simulink model "latest_coil"  (R2021b)
settings: Solver=FixedStepAuto  StartTime=-18e-3  StopTime=50e-3  FixedStep=1e-4  RelTol=1e-3
undefined symbols (not defined in the file): X, Y, Z
libraries: sm_lib x28, nesl_utility x9
(part 2 of 5)

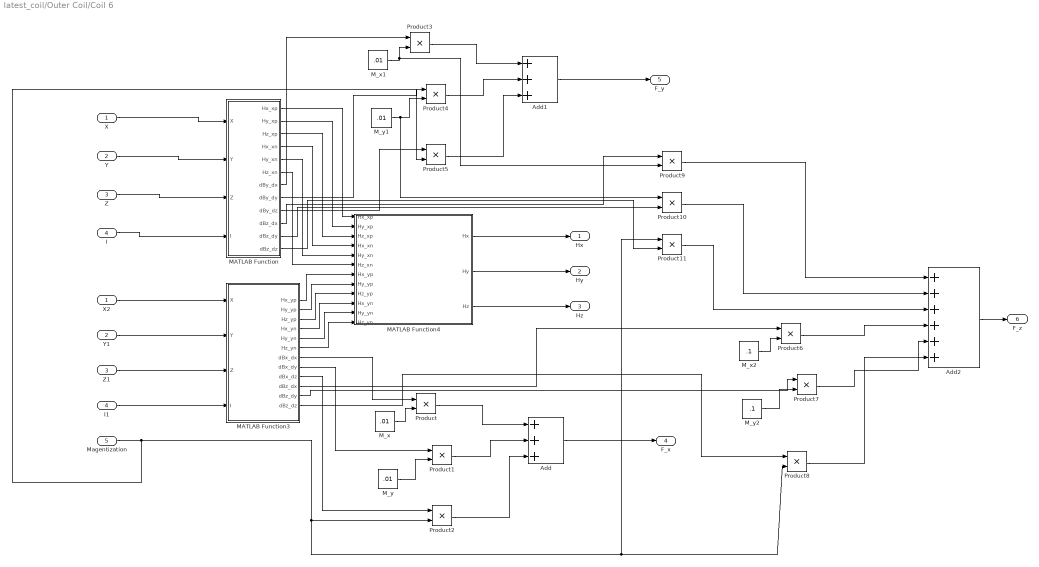
== system latest_coil/Outer Coil/Coil 6 ==
  X : Inport
  Y : Inport  Port=2
  Z : Inport  Port=3
  I : Inport  Port=4
  Magentization : Inport  Port=5
  Add : Sum  Inputs=+++
  Add1 : Sum  Inputs=+++
  Add2 : Sum  Inputs=++++++
  I1 : InportShadow  Port=4
  MATLAB Function : MATLAB Function  TreatAsAtomicUnit=on
  MATLAB Function3 : MATLAB Function  TreatAsAtomicUnit=on
  MATLAB Function4 : MATLAB Function  TreatAsAtomicUnit=on
  M_x : Constant  Value=.01
  M_x1 : Constant  Value=.01
  M_x2 : Constant  Value=.1
  M_y : Constant  Value=.01
  M_y1 : Constant  Value=.01
  M_y2 : Constant  Value=.1
  Product{,1..11} (12 alike) : Product
  X2 : InportShadow
  Y1 : InportShadow  Port=2
  Z1 : InportShadow  Port=3
  Hx : Outport
  Hy : Outport  Port=2
  Hz : Outport  Port=3
  F_x : Outport  Port=4
  F_y : Outport  Port=5
  F_z : Outport  Port=6
  wires:
  Add2/1 -> F_z/1
  Product11/1 -> Add2/3
  Product10/1 -> Add2/2
  Product9/1 -> Add2/1
  MATLAB Function/12(dBz_dz) -> Product11/2
  MATLAB Function/11(dBz_dy) -> Product10/2
  MATLAB Function/10(dBz_dx) -> Product9/1
  MATLAB Function/8(dBy_dy) -> Product4/1
  M_x1/1 -> Product3/2, Product9/2
  MATLAB Function3/12(dBz_dz) -> Product8/1
  Product8/1 -> Add2/6
  M_x2/1 -> Product6/2
  MATLAB Function3/10(dBz_dx) -> Product6/1
  MATLAB Function3/11(dBz_dy) -> Product7/1
  M_y2/1 -> Product7/2
  Product6/1 -> Add2/4
  Product7/1 -> Add2/5
  MATLAB Function/7(dBy_dx) -> Product3/1
  M_y1/1 -> Product4/2, Product10/1
  MATLAB Function/9(dBy_dz) -> Product5/1
  Magentization/1 -> Product5/2, Product8/2, Product11/1, Product2/2
  Product3/1 -> Add1/1
  Product4/1 -> Add1/2
  Product5/1 -> Add1/3
  Add1/1 -> F_y/1
  Add/1 -> F_x/1
  Product2/1 -> Add/3
  Product1/1 -> Add/2
  Product/1 -> Add/1
  MATLAB Function3/9(dBx_dz) -> Product2/1
  M_y/1 -> Product1/2
  MATLAB Function3/8(dBx_dy) -> Product1/1
  MATLAB Function3/7(dBx_dx) -> Product/1
  M_x/1 -> Product/2
  Z1/1 -> MATLAB Function3/3(Z)
  Y1/1 -> MATLAB Function3/2(Y)
  X2/1 -> MATLAB Function3/1(X)
  I/1 -> MATLAB Function/4(I)
  MATLAB Function/2(Hy_xp) -> MATLAB Function4/2(Hy_xp)
  MATLAB Function3/6(Hz_yn) -> MATLAB Function4/12(Hz_yn)
  MATLAB Function3/5(Hy_yn) -> MATLAB Function4/11(Hy_yn)
  MATLAB Function/5(Hy_xn) -> MATLAB Function4/5(Hy_xn)
  Y/1 -> MATLAB Function/2(Y)
  MATLAB Function3/2(Hy_yp) -> MATLAB Function4/8(Hy_yp)
  MATLAB Function/1(Hx_xp) -> MATLAB Function4/1(Hx_xp)
  MATLAB Function/4(Hx_xn) -> MATLAB Function4/4(Hx_xn)
  MATLAB Function3/3(Hz_yp) -> MATLAB Function4/9(Hz_yp)
  MATLAB Function3/4(Hx_yn) -> MATLAB Function4/10(Hx_yn)
  MATLAB Function3/1(Hx_yp) -> MATLAB Function4/7(Hx_yp)
  MATLAB Function4/2(Hy) -> Hy/1
  MATLAB Function/3(Hz_xp) -> MATLAB Function4/3(Hz_xp)
  Z/1 -> MATLAB Function/3(Z)
  MATLAB Function/6(Hz_xn) -> MATLAB Function4/6(Hz_xn)
  I1/1 -> MATLAB Function3/4(I)
  MATLAB Function4/1(Hx) -> Hx/1
  X/1 -> MATLAB Function/1(X)
  MATLAB Function4/3(Hz) -> Hz/1

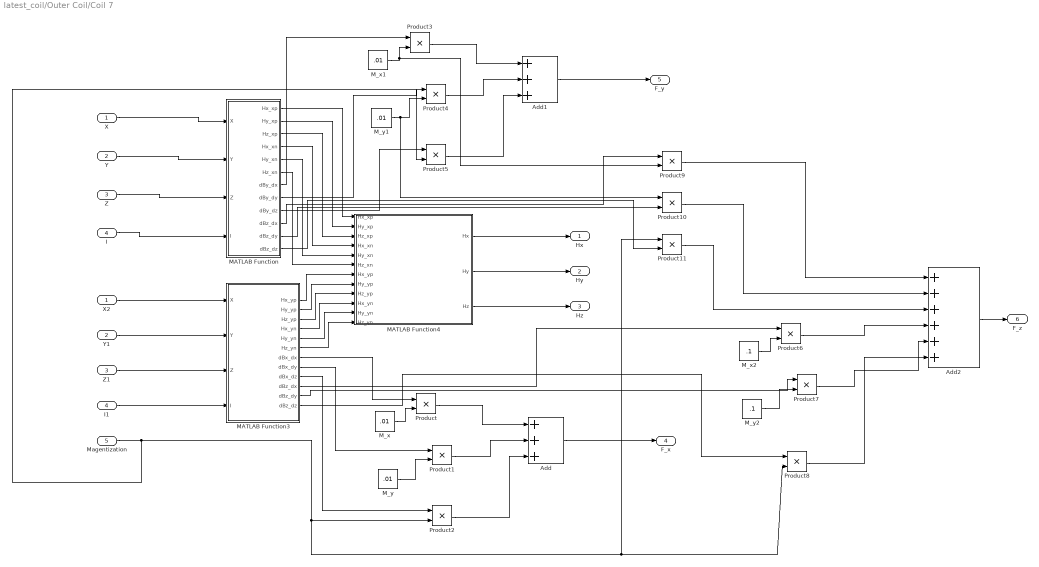
== system latest_coil/Outer Coil/Coil 7 ==
  X : Inport
  Y : Inport  Port=2
  Z : Inport  Port=3
  I : Inport  Port=4
  Magentization : Inport  Port=5
  Add : Sum  Inputs=+++
  Add1 : Sum  Inputs=+++
  Add2 : Sum  Inputs=++++++
  I1 : InportShadow  Port=4
  MATLAB Function : MATLAB Function  TreatAsAtomicUnit=on
  MATLAB Function3 : MATLAB Function  TreatAsAtomicUnit=on
  MATLAB Function4 : MATLAB Function  TreatAsAtomicUnit=on
  M_x : Constant  Value=.01
  M_x1 : Constant  Value=.01
  M_x2 : Constant  Value=.1
  M_y : Constant  Value=.01
  M_y1 : Constant  Value=.01
  M_y2 : Constant  Value=.1
  Product{,1..11} (12 alike) : Product
  X2 : InportShadow
  Y1 : InportShadow  Port=2
  Z1 : InportShadow  Port=3
  Hx : Outport
  Hy : Outport  Port=2
  Hz : Outport  Port=3
  F_x : Outport  Port=4
  F_y : Outport  Port=5
  F_z : Outport  Port=6
  wires:
  MATLAB Function4/3(Hz) -> Hz/1
  X/1 -> MATLAB Function/1(X)
  MATLAB Function4/1(Hx) -> Hx/1
  I1/1 -> MATLAB Function3/4(I)
  MATLAB Function/6(Hz_xn) -> MATLAB Function4/6(Hz_xn)
  Z/1 -> MATLAB Function/3(Z)
  MATLAB Function/3(Hz_xp) -> MATLAB Function4/3(Hz_xp)
  MATLAB Function4/2(Hy) -> Hy/1
  MATLAB Function3/1(Hx_yp) -> MATLAB Function4/7(Hx_yp)
  MATLAB Function3/4(Hx_yn) -> MATLAB Function4/10(Hx_yn)
  MATLAB Function3/3(Hz_yp) -> MATLAB Function4/9(Hz_yp)
  MATLAB Function/4(Hx_xn) -> MATLAB Function4/4(Hx_xn)
  MATLAB Function/1(Hx_xp) -> MATLAB Function4/1(Hx_xp)
  MATLAB Function3/2(Hy_yp) -> MATLAB Function4/8(Hy_yp)
  Y/1 -> MATLAB Function/2(Y)
  MATLAB Function/5(Hy_xn) -> MATLAB Function4/5(Hy_xn)
  MATLAB Function3/5(Hy_yn) -> MATLAB Function4/11(Hy_yn)
  MATLAB Function3/6(Hz_yn) -> MATLAB Function4/12(Hz_yn)
  MATLAB Function/2(Hy_xp) -> MATLAB Function4/2(Hy_xp)
  I/1 -> MATLAB Function/4(I)
  X2/1 -> MATLAB Function3/1(X)
  Y1/1 -> MATLAB Function3/2(Y)
  Z1/1 -> MATLAB Function3/3(Z)
  M_x/1 -> Product/2
  MATLAB Function3/7(dBx_dx) -> Product/1
  MATLAB Function3/8(dBx_dy) -> Product1/1
  M_y/1 -> Product1/2
  MATLAB Function3/9(dBx_dz) -> Product2/1
  Product/1 -> Add/1
  Product1/1 -> Add/2
  Product2/1 -> Add/3
  Add/1 -> F_x/1
  Add1/1 -> F_y/1
  Product5/1 -> Add1/3
  Product4/1 -> Add1/2
  Product3/1 -> Add1/1
  Magentization/1 -> Product2/2, Product11/1, Product8/2, Product5/2
  MATLAB Function/9(dBy_dz) -> Product5/1
  M_y1/1 -> Product10/1, Product4/2
  MATLAB Function/7(dBy_dx) -> Product3/1
  Product7/1 -> Add2/5
  Product6/1 -> Add2/4
  M_y2/1 -> Product7/2
  MATLAB Function3/11(dBz_dy) -> Product7/1
  MATLAB Function3/10(dBz_dx) -> Product6/1
  M_x2/1 -> Product6/2
  Product8/1 -> Add2/6
  MATLAB Function3/12(dBz_dz) -> Product8/1
  M_x1/1 -> Product9/2, Product3/2
  MATLAB Function/8(dBy_dy) -> Product4/1
  MATLAB Function/10(dBz_dx) -> Product9/1
  MATLAB Function/11(dBz_dy) -> Product10/2
  MATLAB Function/12(dBz_dz) -> Product11/2
  Product9/1 -> Add2/1
  Product10/1 -> Add2/2
  Product11/1 -> Add2/3
  Add2/1 -> F_z/1

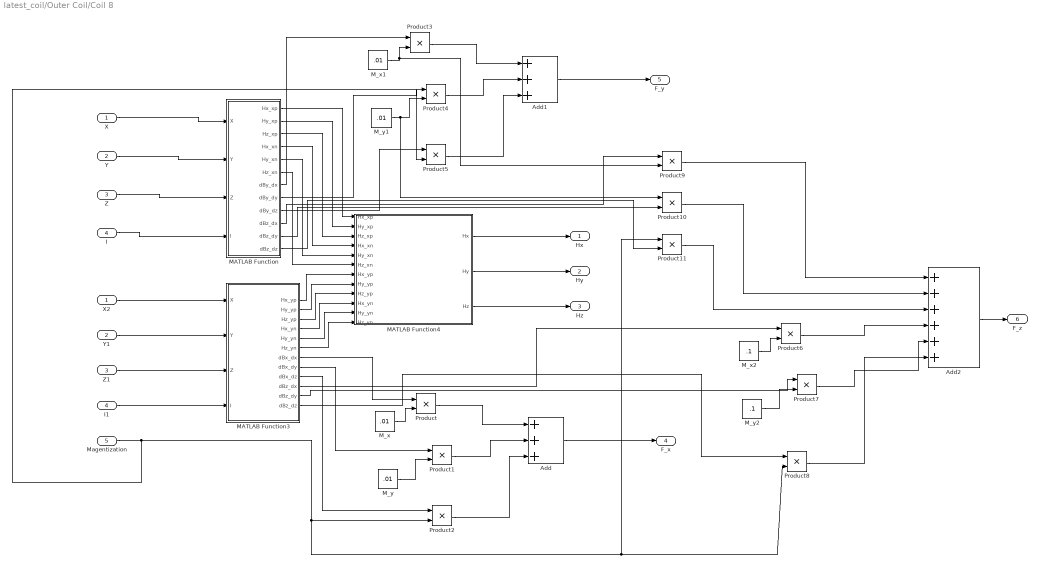
== system latest_coil/Outer Coil/Coil 8 ==
  X : Inport
  Y : Inport  Port=2
  Z : Inport  Port=3
  I : Inport  Port=4
  Magentization : Inport  Port=5
  Add : Sum  Inputs=+++
  Add1 : Sum  Inputs=+++
  Add2 : Sum  Inputs=++++++
  I1 : InportShadow  Port=4
  MATLAB Function : MATLAB Function  TreatAsAtomicUnit=on
  MATLAB Function3 : MATLAB Function  TreatAsAtomicUnit=on
  MATLAB Function4 : MATLAB Function  TreatAsAtomicUnit=on
  M_x : Constant  Value=.01
  M_x1 : Constant  Value=.01
  M_x2 : Constant  Value=.1
  M_y : Constant  Value=.01
  M_y1 : Constant  Value=.01
  M_y2 : Constant  Value=.1
  Product{,1..11} (12 alike) : Product
  X2 : InportShadow
  Y1 : InportShadow  Port=2
  Z1 : InportShadow  Port=3
  Hx : Outport
  Hy : Outport  Port=2
  Hz : Outport  Port=3
  F_x : Outport  Port=4
  F_y : Outport  Port=5
  F_z : Outport  Port=6
  wires:
  MATLAB Function4/3(Hz) -> Hz/1
  X/1 -> MATLAB Function/1(X)
  MATLAB Function4/1(Hx) -> Hx/1
  I1/1 -> MATLAB Function3/4(I)
  MATLAB Function/6(Hz_xn) -> MATLAB Function4/6(Hz_xn)
  Z/1 -> MATLAB Function/3(Z)
  MATLAB Function/3(Hz_xp) -> MATLAB Function4/3(Hz_xp)
  MATLAB Function4/2(Hy) -> Hy/1
  MATLAB Function3/1(Hx_yp) -> MATLAB Function4/7(Hx_yp)
  MATLAB Function3/4(Hx_yn) -> MATLAB Function4/10(Hx_yn)
  MATLAB Function3/3(Hz_yp) -> MATLAB Function4/9(Hz_yp)
  MATLAB Function/4(Hx_xn) -> MATLAB Function4/4(Hx_xn)
  MATLAB Function/1(Hx_xp) -> MATLAB Function4/1(Hx_xp)
  MATLAB Function3/2(Hy_yp) -> MATLAB Function4/8(Hy_yp)
  Y/1 -> MATLAB Function/2(Y)
  MATLAB Function/5(Hy_xn) -> MATLAB Function4/5(Hy_xn)
  MATLAB Function3/5(Hy_yn) -> MATLAB Function4/11(Hy_yn)
  MATLAB Function3/6(Hz_yn) -> MATLAB Function4/12(Hz_yn)
  MATLAB Function/2(Hy_xp) -> MATLAB Function4/2(Hy_xp)
  I/1 -> MATLAB Function/4(I)
  X2/1 -> MATLAB Function3/1(X)
  Y1/1 -> MATLAB Function3/2(Y)
  Z1/1 -> MATLAB Function3/3(Z)
  M_x/1 -> Product/2
  MATLAB Function3/7(dBx_dx) -> Product/1
  MATLAB Function3/8(dBx_dy) -> Product1/1
  M_y/1 -> Product1/2
  MATLAB Function3/9(dBx_dz) -> Product2/1
  Product/1 -> Add/1
  Product1/1 -> Add/2
  Product2/1 -> Add/3
  Add/1 -> F_x/1
  Add1/1 -> F_y/1
  Product5/1 -> Add1/3
  Product4/1 -> Add1/2
  Product3/1 -> Add1/1
  Magentization/1 -> Product2/2, Product11/1, Product8/2, Product5/2
  MATLAB Function/9(dBy_dz) -> Product5/1
  M_y1/1 -> Product10/1, Product4/2
  MATLAB Function/7(dBy_dx) -> Product3/1
  Product7/1 -> Add2/5
  Product6/1 -> Add2/4
  M_y2/1 -> Product7/2
  MATLAB Function3/11(dBz_dy) -> Product7/1
  MATLAB Function3/10(dBz_dx) -> Product6/1
  M_x2/1 -> Product6/2
  Product8/1 -> Add2/6
  MATLAB Function3/12(dBz_dz) -> Product8/1
  M_x1/1 -> Product9/2, Product3/2
  MATLAB Function/8(dBy_dy) -> Product4/1
  MATLAB Function/10(dBz_dx) -> Product9/1
  MATLAB Function/11(dBz_dy) -> Product10/2
  MATLAB Function/12(dBz_dz) -> Product11/2
  Product9/1 -> Add2/1
  Product10/1 -> Add2/2
  Product11/1 -> Add2/3
  Add2/1 -> F_z/1

== system latest_coil/Outer Coil/Coil 9 ==
  X : Inport
  Y : Inport  Port=2
  Z : Inport  Port=3
  I : Inport  Port=4
  Magentization : Inport  Port=5
  Add : Sum  Inputs=+++
  Add1 : Sum  Inputs=+++
  Add2 : Sum  Inputs=++++++
  I1 : InportShadow  Port=4
  MATLAB Function : MATLAB Function  TreatAsAtomicUnit=on
  MATLAB Function3 : MATLAB Function  TreatAsAtomicUnit=on
  MATLAB Function4 : MATLAB Function  TreatAsAtomicUnit=on
  M_x : Constant  Value=.01
  M_x1 : Constant  Value=.01
  M_x2 : Constant  Value=.1
  M_y : Constant  Value=.01
  M_y1 : Constant  Value=.01
  M_y2 : Constant  Value=.1
  Product{,1..11} (12 alike) : Product
  X2 : InportShadow
  Y1 : InportShadow  Port=2
  Z1 : InportShadow  Port=3
  Hx : Outport
  Hy : Outport  Port=2
  Hz : Outport  Port=3
  F_x : Outport  Port=4
  F_y : Outport  Port=5
  F_z : Outport  Port=6
  wires:
  Add2/1 -> F_z/1
  Product11/1 -> Add2/3
  Product10/1 -> Add2/2
  Product9/1 -> Add2/1
  MATLAB Function/12(dBz_dz) -> Product11/2
  MATLAB Function/11(dBz_dy) -> Product10/2
  MATLAB Function/10(dBz_dx) -> Product9/1
  MATLAB Function/8(dBy_dy) -> Product4/1
  M_x1/1 -> Product3/2, Product9/2
  MATLAB Function3/12(dBz_dz) -> Product8/1
  Product8/1 -> Add2/6
  M_x2/1 -> Product6/2
  MATLAB Function3/10(dBz_dx) -> Product6/1
  MATLAB Function3/11(dBz_dy) -> Product7/1
  M_y2/1 -> Product7/2
  Product6/1 -> Add2/4
  Product7/1 -> Add2/5
  MATLAB Function/7(dBy_dx) -> Product3/1
  M_y1/1 -> Product4/2, Product10/1
  MATLAB Function/9(dBy_dz) -> Product5/1
  Magentization/1 -> Product5/2, Product8/2, Product11/1, Product2/2
  Product3/1 -> Add1/1
  Product4/1 -> Add1/2
  Product5/1 -> Add1/3
  Add1/1 -> F_y/1
  Add/1 -> F_x/1
  Product2/1 -> Add/3
  Product1/1 -> Add/2
  Product/1 -> Add/1
  MATLAB Function3/9(dBx_dz) -> Product2/1
  M_y/1 -> Product1/2
  MATLAB Function3/8(dBx_dy) -> Product1/1
  MATLAB Function3/7(dBx_dx) -> Product/1
  M_x/1 -> Product/2
  Z1/1 -> MATLAB Function3/3(Z)
  Y1/1 -> MATLAB Function3/2(Y)
  X2/1 -> MATLAB Function3/1(X)
  I/1 -> MATLAB Function/4(I)
  MATLAB Function/2(Hy_xp) -> MATLAB Function4/2(Hy_xp)
  MATLAB Function3/6(Hz_yn) -> MATLAB Function4/12(Hz_yn)
  MATLAB Function3/5(Hy_yn) -> MATLAB Function4/11(Hy_yn)
  MATLAB Function/5(Hy_xn) -> MATLAB Function4/5(Hy_xn)
  Y/1 -> MATLAB Function/2(Y)
  MATLAB Function3/2(Hy_yp) -> MATLAB Function4/8(Hy_yp)
  MATLAB Function/1(Hx_xp) -> MATLAB Function4/1(Hx_xp)
  MATLAB Function/4(Hx_xn) -> MATLAB Function4/4(Hx_xn)
  MATLAB Function3/3(Hz_yp) -> MATLAB Function4/9(Hz_yp)
  MATLAB Function3/4(Hx_yn) -> MATLAB Function4/10(Hx_yn)
  MATLAB Function3/1(Hx_yp) -> MATLAB Function4/7(Hx_yp)
  MATLAB Function4/2(Hy) -> Hy/1
  MATLAB Function/3(Hz_xp) -> MATLAB Function4/3(Hz_xp)
  Z/1 -> MATLAB Function/3(Z)
  MATLAB Function/6(Hz_xn) -> MATLAB Function4/6(Hz_xn)
  I1/1 -> MATLAB Function3/4(I)
  MATLAB Function4/1(Hx) -> Hx/1
  X/1 -> MATLAB Function/1(X)
  MATLAB Function4/3(Hz) -> Hz/1

== matlab function latest_coil/Inner Coil/Coil 2/MATLAB Function3 ==
  data: X input; Hx_yp output; Y input; Z input; I input; Hy_yp output; Hz_yp output; Hx_yn output; Hy_yn output; Hz_yn output; dBx_dx output; dBx_dy output; dBx_dz output; dBz_dx output; dBz_dy output; dBz_dz output
function [Hx_yp, Hy_yp, Hz_yp, Hx_yn, Hy_yn, Hz_yn, dBx_dx, dBx_dy, dBx_dz, dBz_dx, dBz_dy, dBz_dz] = field_y(X, Y, Z, I)

n = 2;
gy = 460e-6;
% gx = 1.075e-3;
gz = 0;

m0 = 4*pi*1e-7;
k = 0.4e-3;
yp1 = -0.6e-3 - (n-1)*k;
yp2 = 0.6e-3 + (n-1)*k;
a_xp = gy;
a_zp = gz;
k_yp = 1./(4*pi*((a_xp-X).^2+(a_zp-Z).^2));
kyp = (yp2-Y)./((yp2-Y).^2+(a_xp-X).^2+(a_zp-Z).^2).^0.5;
k_2yp = (yp1-Y)./((yp1-Y).^2+(a_xp-X).^2+(a_zp-Z).^2).^0.5;

Hx_yp = -((a_zp-Z).*k_yp.*(kyp - k_2yp))*I*m0;
Hy_yp = zeros(size(X,1),size(Y,1),size(Z,1));
Hz_yp = (-(a_xp-X).*k_yp.*(kyp - k_2yp))*I*m0;

a_xn = -gy;
yn1 = -0.8e-3 - (n-1)*k;
yn2 = 0.8e-3 + (n-1)*k;
k_yn = 1./(4*pi*((a_xn-X).^2+(a_zp-Z).^2));
kyn = (yn2-Y)./((yn2-Y).^2+(a_xn-X).^2+(a_zp-Z).^2).^0.5;
k_2yn = (yn1-Y)./((yn1-Y).^2+(a_xn-X).^2+(a_zp-Z).^2).^0.5;

Hx_yn = ((a_zp-Z).*k_yn.*(kyn - k_2yn))*I*m0;
Hy_yn = zeros(size(X,1),size(Y,1),size(Z,1));
Hz_yn = ((a_xn-X).*k_yn.*(kyn - k_2yn))*I*m0;

dBxn_dx = - (I*Z*m0*(((Y - yn1)*(2*X - 2*a_xn))/(2*((X - a_xn)^2 + (Z - a_zp)^2 + (Y - yn1)^2)^(3/2)) - ((Y - yn2)*(2*X - 2*a_xn))/(2*((X - a_xn)^2 + (Z - a_zp)^2 + (Y - yn2)^2)^(3/2))))/(4*pi*((X - a_xn)^2 + (Z - a_zp)^2)) - (I*Z*m0*((Y - yn1)/((X - a_xn)^2 + (Z - a_zp)^2 + (Y - yn1)^2)^(1/2) - (Y - yn2)/((X - a_xn)^2 + (Z - a_zp)^2 + (Y - yn2)^2)^(1/2))*(2*X - 2*a_xn))/(4*pi*((X - a_xn)^2 + (Z - a_zp)^2)^2);
dBxp_dx = (I*Z*m0*(((Y - yp1)*(2*X - 2*a_xp))/(2*((X - a_xp)^2 + (Z - a_zp)^2 + (Y - yp1)^2)^(3/2)) - ((Y - yp2)*(2*X - 2*a_xp))/(2*((X - a_xp)^2 + (Z - a_zp)^2 + (Y - yp2)^2)^(3/2))))/(4*pi*((X - a_xp)^2 + (Z - a_zp)^2)) + (I*Z*m0*((Y - yp1)/((X - a_xp)^2 + (Z - a_zp)^2 + (Y - yp1)^2)^(1/2) - (Y - yp2)/((X - a_xp)^2 + (Z - a_zp)^2 + (Y - yp2)^2)^(1/2))*(2*X - 2*a_xp))/(4*pi*((X - a_xp)^2 + (Z - a_zp)^2)^2);
dBx_dx = dBxp_dx + dBxn_dx;

dBxp_dy = -(I*Z*m0*(1/((X - a_xp)^2 + (Z - a_zp)^2 + (Y - yp1)^2)^(1/2) - 1/((X - a_xp)^2 + (Z - a_zp)^2 + (Y - yp2)^2)^(1/2) - ((Y - yp1)*(2*Y - 2*yp1))/(2*((X - a_xp)^2 + (Z - a_zp)^2 + (Y - yp1)^2)^(3/2)) + ((Y - yp2)*(2*Y - 2*yp2))/(2*((X - a_xp)^2 + (Z - a_zp)^2 + (Y - yp2)^2)^(3/2))))/(4*pi*((X - a_xp)^2 + (Z - a_zp)^2));
dBxn_dy = (I*Z*m0*(1/((X - a_xn)^2 + (Z - a_zp)^2 + (Y - yn1)^2)^(1/2) - 1/((X - a_xn)^2 + (Z - a_zp)^2 + (Y - yn2)^2)^(1/2) - ((Y - yn1)*(2*Y - 2*yn1))/(2*((X - a_xn)^2 + (Z - a_zp)^2 + (Y - yn1)^2)^(3/2)) + ((Y - yn2)*(2*Y - 2*yn2))/(2*((X - a_xn)^2 + (Z - a_zp)^2 + (Y - yn2)^2)^(3/2))))/(4*pi*((X - a_xn)^2 + (Z - a_zp)^2));
dBx_dy = dBxp_dy + dBxn_dy;

dBxp_dz = (I*Z*m0*(((Y - yp1)*(2*Z - 2*a_zp))/(2*((X - a_xp)^2 + (Z - a_zp)^2 + (Y - yp1)^2)^(3/2)) - ((Y - yp2)*(2*Z - 2*a_zp))/(2*((X - a_xp)^2 + (Z - a_zp)^2 + (Y - yp2)^2)^(3/2))))/(4*pi*((X - a_xp)^2 + (Z - a_zp)^2)) - (I*m0*((Y - yp1)/((X - a_xp)^2 + (Z - a_zp)^2 + (Y - yp1)^2)^(1/2) - (Y - yp2)/((X - a_xp)^2 + (Z - a_zp)^2 + (Y - yp2)^2)^(1/2)))/(4*pi*((X - a_xp)^2 + (Z - a_zp)^2)) + (I*Z*m0*((Y - yp1)/((X - a_xp)^2 + (Z - a_zp)^2 + (Y - yp1)^2)^(1/2) - (Y - yp2)/((X - a_xp)^2 + (Z - a_zp)^2 + (Y - yp2)^2)^(1/2))*(2*Z - 2*a_zp))/(4*pi*((X - a_xp)^2 + (Z - a_zp)^2)^2);
dBxn_dz = (I*m0*((Y - yn1)/((X - a_xn)^2 + (Z - a_zp)^2 + (Y - yn1)^2)^(1/2) - (Y - yn2)/((X - a_xn)^2 + (Z - a_zp)^2 + (Y - yn2)^2)^(1/2)))/(4*pi*((X - a_xn)^2 + (Z - a_zp)^2)) - (I*Z*m0*(((Y - yn1)*(2*Z - 2*a_zp))/(2*((X - a_xn)^2 + (Z - a_zp)^2 + (Y - yn1)^2)^(3/2)) - ((Y - yn2)*(2*Z - 2*a_zp))/(2*((X - a_xn)^2 + (Z - a_zp)^2 + (Y - yn2)^2)^(3/2))))/(4*pi*((X - a_xn)^2 + (Z - a_zp)^2)) - (I*Z*m0*((Y - yn1)/((X - a_xn)^2 + (Z - a_zp)^2 + (Y - yn1)^2)^(1/2) - (Y - yn2)/((X - a_xn)^2 + (Z - a_zp)^2 + (Y - yn2)^2)^(1/2))*(2*Z - 2*a_zp))/(4*pi*((X - a_xn)^2 + (Z - a_zp)^2)^2);
dBx_dz = dBxp_dz + dBxn_dz;

dBzn_dx = (I*m0*(X - a_xn)*(((Y - yn1)*(2*X - 2*a_xn))/(2*((X - a_xn)^2 + (Z - a_zp)^2 + (Y - yn1)^2)^(3/2)) - ((Y - yn2)*(2*X - 2*a_xn))/(2*((X - a_xn)^2 + (Z - a_zp)^2 + (Y - yn2)^2)^(3/2))))/(4*pi*(Z^2 + (X - a_xn)^2)) - (I*m0*((Y - yn1)/((X - a_xn)^2 + (Z - a_zp)^2 + (Y - yn1)^2)^(1/2) - (Y - yn2)/((X - a_xn)^2 + (Z - a_zp)^2 + (Y - yn2)^2)^(1/2)))/(4*pi*(Z^2 + (X - a_xn)^2)) + (I*m0*((Y - yn1)/((X - a_xn)^2 + (Z - a_zp)^2 + (Y - yn1)^2)^(1/2) - (Y - yn2)/((X - a_xn)^2 + (Z - a_zp)^2 + (Y - yn2)^2)^(1/2))*(X - a_xn)*(2*X - 2*a_xn))/(4*pi*(Z^2 + (X - a_xn)^2)^2);
dBzp_dx = (I*m0*((Y - yp1)/((X - a_xp)^2 + (Z - a_zp)^2 + (Y - yp1)^2)^(1/2) - (Y - yp2)/((X - a_xp)^2 + (Z - a_zp)^2 + (Y - yp2)^2)^(1/2)))/(4*pi*(Z^2 + (X - a_xp)^2)) - (I*m0*(X - a_xp)*(((Y - yp1)*(2*X - 2*a_xp))/(2*((X - a_xp)^2 + (Z - a_zp)^2 + (Y - yp1)^2)^(3/2)) - ((Y - yp2)*(2*X - 2*a_xp))/(2*((X - a_xp)^2 + (Z - a_zp)^2 + (Y - yp2)^2)^(3/2))))/(4*pi*(Z^2 + (X - a_xp)^2)) - (I*m0*((Y - yp1)/((X - a_xp)^2 + (Z - a_zp)^2 + (Y - yp1)^2)^(1/2) - (Y - yp2)/((X - a_xp)^2 + (Z - a_zp)^2 + (Y - yp2)^2)^(1/2))*(X - a_xp)*(2*X - 2*a_xp))/(4*pi*(Z^2 + (X - a_xp)^2)^2);
dBz_dx = dBzp_dx + dBzn_dx;

dBzn_dy = -(I*m0*(X - a_xn)*(1/((X - a_xn)^2 + (Z - a_zp)^2 + (Y - yn1)^2)^(1/2) - 1/((X - a_xn)^2 + (Z - a_zp)^2 + (Y - yn2)^2)^(1/2) - ((Y - yn1)*(2*Y - 2*yn1))/(2*((X - a_xn)^2 + (Z - a_zp)^2 + (Y - yn1)^2)^(3/2)) + ((Y - yn2)*(2*Y - 2*yn2))/(2*((X - a_xn)^2 + (Z - a_zp)^2 + (Y - yn2)^2)^(3/2))))/(4*pi*(Z^2 + (X - a_xn)^2));
dBzp_dy = (I*m0*(X - a_xp)*(1/((X - a_xp)^2 + (Z - a_zp)^2 + (Y - yp1)^2)^(1/2) - 1/((X - a_xp)^2 + (Z - a_zp)^2 + (Y - yp2)^2)^(1/2) - ((Y - yp1)*(2*Y - 2*yp1))/(2*((X - a_xp)^2 + (Z - a_zp)^2 + (Y - yp1)^2)^(3/2)) + ((Y - yp2)*(2*Y - 2*yp2))/(2*((X - a_xp)^2 + (Z - a_zp)^2 + (Y - yp2)^2)^(3/2))))/(4*pi*(Z^2 + (X - a_xp)^2));
dBz_dy = dBzn_dy + dBzp_dy;

dBzn_dz = (I*m0*(X - a_xn)*(((Y - yn1)*(2*Z - 2*a_zp))/(2*((X - a_xn)^2 + (Z - a_zp)^2 + (Y - yn1)^2)^(3/2)) - ((Y - yn2)*(2*Z - 2*a_zp))/(2*((X - a_xn)^2 + (Z - a_zp)^2 + (Y - yn2)^2)^(3/2))))/(4*pi*(Z^2 + (X - a_xn)^2)) + (I*Z*m0*((Y - yn1)/((X - a_xn)^2 + (Z - a_zp)^2 + (Y - yn1)^2)^(1/2) - (Y - yn2)/((X - a_xn)^2 + (Z - a_zp)^2 + (Y - yn2)^2)^(1/2))*(X - a_xn))/(2*pi*(Z^2 + (X - a_xn)^2)^2);
dBzp_dz = - (I*m0*(X - a_xp)*(((Y - yp1)*(2*Z - 2*a_zp))/(2*((X - a_xp)^2 + (Z - a_zp)^2 + (Y - yp1)^2)^(3/2)) - ((Y - yp2)*(2*Z - 2*a_zp))/(2*((X - a_xp)^2 + (Z - a_zp)^2 + (Y - yp2)^2)^(3/2))))/(4*pi*(Z^2 + (X - a_xp)^2)) - (I*Z*m0*((Y - yp1)/((X - a_xp)^2 + (Z - a_zp)^2 + (Y - yp1)^2)^(1/2) - (Y - yp2)/((X - a_xp)^2 + (Z - a_zp)^2 + (Y - yp2)^2)^(1/2))*(X - a_xp))/(2*pi*(Z^2 + (X - a_xp)^2)^2);
dBz_dz = dBzn_dz + dBzp_dz;
end

== matlab function latest_coil/Inner Coil/Coil 2/MATLAB Function4 ==
  data: Hx_xp input; Hy_xp input; Hz_xp input; Hx output; Hx_xn input; Hy_xn input; Hy output; Hz output; Hz_xn input; Hx_yp input; Hy_yp input; Hz_yp input; Hx_yn input; Hy_yn input; Hz_yn input
function [Hx, Hy, Hz] = field_sum(Hx_xp, Hy_xp, Hz_xp, Hx_xn, Hy_xn, Hz_xn, Hx_yp, Hy_yp, Hz_yp, Hx_yn, Hy_yn, Hz_yn)
Hx = Hx_xp + Hx_xn + Hx_yp + Hx_yn;
Hy = Hy_xp + Hy_xn + Hy_yp + Hy_yn;
Hz = Hz_xp + Hz_xn + Hz_yp + Hz_yn;
end

== matlab function latest_coil/MATLAB Function1 ==
  data: Ff_y output; Fext_y input; vy input
function Ff_y = friction(Fext_y,vy)
Coeff_of_Fric = 0.432;
g = 9.8;
mass_of_bot = 9.17345e-05;

% if  Fext_y < 0 && vy >= 0 %When force is in negative direction and velocity is in positive direction (impossible case) (Removing this case implies object doesn't move)
%     Ff_y = 0;
% elseif  Fext_y > 0 && vy <= 0 %When force is in positivedirection and velocity is in positive direction (impossible case)
%     Ff_y = 0;
% elseif  vy < 0 %When velocity is in negative direction friction is positive (Object is moving)
%     Ff_y = Coeff_of_Fric*mass_of_bot*g;
% elseif  vy > 0 %When velocity is in positive direction friction is negative (Object is moving)
%     Ff_y = -Coeff_of_Fric*mass_of_bot*g;
% elseif (abs(Fext_y) >= Coeff_of_Fric*mass_of_bot*g  &&  vy < 0 ) || (abs(Fext_y) >= Coeff_of_Fric*mass_of_bot*g && vy > 0) %When applied force greater than couloumb friction and 
%                                                                                                                        % moves is positive or negative direction, then Couloumb friction opposes that motion
%     Ff_y = -Coeff_of_Fric*mass_of_bot*g*sign(Fext_y);
% 
% elseif (abs(Fext_y) < Coeff_of_Fric*mass_of_bot*g && Fext_y~= 0) %When applied force less than Coloumb Friction but not equal to zero, Friction force is applied force
%     Ff_y = -Fext_y;
% else %When applied force is zero or when object not moving
%     Ff_y = -Fext_y;
% end

if abs(vy)<0.01
    if abs(Fext_y)>Coeff_of_Fric*mass_of_bot*g
        Ff_y=-Coeff_of_Fric*mass_of_bot*g*sign(Fext_y);
    else
        Ff_y=-Fext_y-vy;
    end
else
    Ff_y=-Coeff_of_Fric*mass_of_bot*g*sign(vy);
end

== matlab function latest_coil/Inner Coil/Coil 3/MATLAB Function ==
  data: X input; Hx_xp output; Y input; Z input; I input; Hy_xp output; Hz_xp output; Hx_xn output; Hy_xn output; Hz_xn output; dBy_dx output; dBy_dy output; dBy_dz output; dBz_dx output; dBz_dy output; dBz_dz output
function [Hx_xp, Hy_xp, Hz_xp, Hx_xn, Hy_xn, Hz_xn,dBy_dx ,dBy_dy, dBy_dz, dBz_dx ,dBz_dy, dBz_dz] = field_x(X, Y, Z, I)
n = 3;
% gy = 440e-6;
gx = 1.475e-3;
gz = 0;
m0 = 4*pi*1e-7;
k = 0.4e-3;
xp1 = -0.8e-3 - (n-1)*k;
xp2 = 0.8e-3 + (n-1)*k;
a_yp = gx; 
a_zp = gz;
k_p = 1./(4*pi*((a_yp-Y).^2+(a_zp-Z).^2));
kxp = (xp2-X)./((xp2-X).^2+(a_yp-Y).^2+(a_zp-Z).^2).^0.5;
k_2xp = (xp1-X)./((xp1-X).^2+(a_yp-Y).^2+(a_zp-Z).^2).^0.5;

Hx_xp = zeros(size(X,1),size(Y,1),size(Z,1));
Hy_xp = (-(a_zp-Z).*k_p.*(kxp - k_2xp))*I*m0;
Hz_xp = (-(a_yp-Y).*k_p.*(kxp - k_2xp))*I*m0;

a_yn = -gx;
xn1 = -1e-3 - (n-1)*k;
xn2 = 1e-3 + (n-1)*k;
k_n = 1./(4*pi*((a_yn-Y).^2+(a_zp-Z).^2));
kxn = (xn2-X)./((xn2-X).^2+(a_yn-Y).^2+(a_zp-Z).^2).^0.5;
k_2xn = (xn1-X)./((xn1-X).^2+(a_yn-Y).^2+(a_zp-Z).^2).^0.5;

Hx_xn = zeros(size(X,1),size(Y,1),size(Z,1));
Hy_xn = ((a_zp-Z).*k_n.*(kxn - k_2xn))*I*m0;
Hz_xn = ((a_yn-Y).*k_n.*(kxn - k_2xn))*I*m0;

dByn_dx = (I*Z*m0*(1/((Y - a_yn)^2 + (Z - a_zp)^2 + (X - xn1)^2)^(1/2) - 1/((Y - a_yn)^2 + (Z - a_zp)^2 + (X - xn2)^2)^(1/2) - ((X - xn1)*(2*X - 2*xn1))/(2*((Y - a_yn)^2 + (Z - a_zp)^2 + (X - xn1)^2)^(3/2)) + ((X - xn2)*(2*X - 2*xn2))/(2*((Y - a_yn)^2 + (Z - a_zp)^2 + (X - xn2)^2)^(3/2))))/(4*pi*((Y - a_yn)^2 + (Z - a_zp)^2));
dByp_dx = -(I*Z*m0*(1/((Y - a_yp)^2 + (Z - a_zp)^2 + (X - xp1)^2)^(1/2) - 1/((Y - a_yp)^2 + (Z - a_zp)^2 + (X - xp2)^2)^(1/2) - ((X - xp1)*(2*X - 2*xp1))/(2*((Y - a_yp)^2 + (Z - a_zp)^2 + (X - xp1)^2)^(3/2)) + ((X - xp2)*(2*X - 2*xp2))/(2*((Y - a_yp)^2 + (Z - a_zp)^2 + (X - xp2)^2)^(3/2))))/(4*pi*((Y - a_yp)^2 + (Z - a_zp)^2));
dBy_dx = dByp_dx + dByn_dx;

dByp_dy = (I*Z*m0*(((X - xp1)*(2*Y - 2*a_yp))/(2*((Y - a_yp)^2 + (Z - a_zp)^2 + (X - xp1)^2)^(3/2)) - ((X - xp2)*(2*Y - 2*a_yp))/(2*((Y - a_yp)^2 + (Z - a_zp)^2 + (X - xp2)^2)^(3/2))))/(4*pi*((Y - a_yp)^2 + (Z - a_zp)^2)) + (I*Z*m0*(2*Y - 2*a_yp)*((X - xp1)/((Y - a_yp)^2 + (Z - a_zp)^2 + (X - xp1)^2)^(1/2) - (X - xp2)/((Y - a_yp)^2 + (Z - a_zp)^2 + (X - xp2)^2)^(1/2)))/(4*pi*((Y - a_yp)^2 + (Z - a_zp)^2)^2);
dByn_dy = - (I*Z*m0*(((X - xn1)*(2*Y - 2*a_yn))/(2*((Y - a_yn)^2 + (Z - a_zp)^2 + (X - xn1)^2)^(3/2)) - ((X - xn2)*(2*Y - 2*a_yn))/(2*((Y - a_yn)^2 + (Z - a_zp)^2 + (X - xn2)^2)^(3/2))))/(4*pi*((Y - a_yn)^2 + (Z - a_zp)^2)) - (I*Z*m0*(2*Y - 2*a_yn)*((X - xn1)/((Y - a_yn)^2 + (Z - a_zp)^2 + (X - xn1)^2)^(1/2) - (X - xn2)/((Y - a_yn)^2 + (Z - a_zp)^2 + (X - xn2)^2)^(1/2)))/(4*pi*((Y - a_yn)^2 + (Z - a_zp)^2)^2);
dBy_dy = dByp_dy + dByn_dy;

dByp_dz = (I*Z*m0*(((X - xp1)*(2*Z - 2*a_zp))/(2*((Y - a_yp)^2 + (Z - a_zp)^2 + (X - xp1)^2)^(3/2)) - ((X - xp2)*(2*Z - 2*a_zp))/(2*((Y - a_yp)^2 + (Z - a_zp)^2 + (X - xp2)^2)^(3/2))))/(4*pi*((Y - a_yp)^2 + (Z - a_zp)^2)) - (I*m0*((X - xp1)/((Y - a_yp)^2 + (Z - a_zp)^2 + (X - xp1)^2)^(1/2) - (X - xp2)/((Y - a_yp)^2 + (Z - a_zp)^2 + (X - xp2)^2)^(1/2)))/(4*pi*((Y - a_yp)^2 + (Z - a_zp)^2)) + (I*Z*m0*(2*Z - 2*a_zp)*((X - xp1)/((Y - a_yp)^2 + (Z - a_zp)^2 + (X - xp1)^2)^(1/2) - (X - xp2)/((Y - a_yp)^2 + (Z - a_zp)^2 + (X - xp2)^2)^(1/2)))/(4*pi*((Y - a_yp)^2 + (Z - a_zp)^2)^2);
dByn_dz = (I*m0*((X - xn1)/((Y - a_yn)^2 + (Z - a_zp)^2 + (X - xn1)^2)^(1/2) - (X - xn2)/((Y - a_yn)^2 + (Z - a_zp)^2 + (X - xn2)^2)^(1/2)))/(4*pi*((Y - a_yn)^2 + (Z - a_zp)^2)) - (I*Z*m0*(((X - xn1)*(2*Z - 2*a_zp))/(2*((Y - a_yn)^2 + (Z - a_zp)^2 + (X - xn1)^2)^(3/2)) - ((X - xn2)*(2*Z - 2*a_zp))/(2*((Y - a_yn)^2 + (Z - a_zp)^2 + (X - xn2)^2)^(3/2))))/(4*pi*((Y - a_yn)^2 + (Z - a_zp)^2)) - (I*Z*m0*(2*Z - 2*a_zp)*((X - xn1)/((Y - a_yn)^2 + (Z - a_zp)^2 + (X - xn1)^2)^(1/2) - (X - xn2)/((Y - a_yn)^2 + (Z - a_zp)^2 + (X - xn2)^2)^(1/2)))/(4*pi*((Y - a_yn)^2 + (Z - a_zp)^2)^2);
dBy_dz = dByp_dz + dByn_dz;

dBzp_dx = (I*m0*(Y - a_yp)*(1/((Y - a_yp)^2 + (Z - a_zp)^2 + (X - xp1)^2)^(1/2) - 1/((Y - a_yp)^2 + (Z - a_zp)^2 + (X - xp2)^2)^(1/2) - ((X - xp1)*(2*X - 2*xp1))/(2*((Y - a_yp)^2 + (Z - a_zp)^2 + (X - xp1)^2)^(3/2)) + ((X - xp2)*(2*X - 2*xp2))/(2*((Y - a_yp)^2 + (Z - a_zp)^2 + (X - xp2)^2)^(3/2))))/(4*pi*(Z^2 + (Y - a_yp)^2));
dBzn_dx = -(I*m0*(Y - a_yn)*(1/((Y - a_yn)^2 + (Z - a_zp)^2 + (X - xn1)^2)^(1/2) - 1/((Y - a_yn)^2 + (Z - a_zp)^2 + (X - xn2)^2)^(1/2) - ((X - xn1)*(2*X - 2*xn1))/(2*((Y - a_yn)^2 + (Z - a_zp)^2 + (X - xn1)^2)^(3/2)) + ((X - xn2)*(2*X - 2*xn2))/(2*((Y - a_yn)^2 + (Z - a_zp)^2 + (X - xn2)^2)^(3/2))))/(4*pi*(Z^2 + (Y - a_yn)^2));
dBz_dx = dBzp_dx + dBzn_dx;

dBzn_dy = (I*m0*(Y - a_yn)*(((X - xn1)*(2*Y - 2*a_yn))/(2*((Y - a_yn)^2 + (Z - a_zp)^2 + (X - xn1)^2)^(3/2)) - ((X - xn2)*(2*Y - 2*a_yn))/(2*((Y - a_yn)^2 + (Z - a_zp)^2 + (X - xn2)^2)^(3/2))))/(4*pi*(Z^2 + (Y - a_yn)^2)) - (I*m0*((X - xn1)/((Y - a_yn)^2 + (Z - a_zp)^2 + (X - xn1)^2)^(1/2) - (X - xn2)/((Y - a_yn)^2 + (Z - a_zp)^2 + (X - xn2)^2)^(1/2)))/(4*pi*(Z^2 + (Y - a_yn)^2)) + (I*m0*(Y - a_yn)*(2*Y - 2*a_yn)*((X - xn1)/((Y - a_yn)^2 + (Z - a_zp)^2 + (X - xn1)^2)^(1/2) - (X - xn2)/((Y - a_yn)^2 + (Z - a_zp)^2 + (X - xn2)^2)^(1/2)))/(4*pi*(Z^2 + (Y - a_yn)^2)^2);
dBzp_dy = (I*m0*((X - xp1)/((Y - a_yp)^2 + (Z - a_zp)^2 + (X - xp1)^2)^(1/2) - (X - xp2)/((Y - a_yp)^2 + (Z - a_zp)^2 + (X - xp2)^2)^(1/2)))/(4*pi*(Z^2 + (Y - a_yp)^2)) - (I*m0*(Y - a_yp)*(((X - xp1)*(2*Y - 2*a_yp))/(2*((Y - a_yp)^2 + (Z - a_zp)^2 + (X - xp1)^2)^(3/2)) - ((X - xp2)*(2*Y - 2*a_yp))/(2*((Y - a_yp)^2 + (Z - a_zp)^2 + (X - xp2)^2)^(3/2))))/(4*pi*(Z^2 + (Y - a_yp)^2)) - (I*m0*(Y - a_yp)*(2*Y - 2*a_yp)*((X - xp1)/((Y - a_yp)^2 + (Z - a_zp)^2 + (X - xp1)^2)^(1/2) - (X - xp2)/((Y - a_yp)^2 + (Z - a_zp)^2 + (X - xp2)^2)^(1/2)))/(4*pi*(Z^2 + (Y - a_yp)^2)^2);
dBz_dy = dBzn_dy + dBzp_dy;

dBzn_dz = (I*m0*(Y - a_yn)*(((X - xn1)*(2*Z - 2*a_zp))/(2*((Y - a_yn)^2 + (Z - a_zp)^2 + (X - xn1)^2)^(3/2)) - ((X - xn2)*(2*Z - 2*a_zp))/(2*((Y - a_yn)^2 + (Z - a_zp)^2 + (X - xn2)^2)^(3/2))))/(4*pi*(Z^2 + (Y - a_yn)^2)) + (I*Z*m0*(Y - a_yn)*((X - xn1)/((Y - a_yn)^2 + (Z - a_zp)^2 + (X - xn1)^2)^(1/2) - (X - xn2)/((Y - a_yn)^2 + (Z - a_zp)^2 + (X - xn2)^2)^(1/2)))/(2*pi*(Z^2 + (Y - a_yn)^2)^2);
dBzp_dz = - (I*m0*(Y - a_yp)*(((X - xp1)*(2*Z - 2*a_zp))/(2*((Y - a_yp)^2 + (Z - a_zp)^2 + (X - xp1)^2)^(3/2)) - ((X - xp2)*(2*Z - 2*a_zp))/(2*((Y - a_yp)^2 + (Z - a_zp)^2 + (X - xp2)^2)^(3/2))))/(4*pi*(Z^2 + (Y - a_yp)^2)) - (I*Z*m0*(Y - a_yp)*((X - xp1)/((Y - a_yp)^2 + (Z - a_zp)^2 + (X - xp1)^2)^(1/2) - (X - xp2)/((Y - a_yp)^2 + (Z - a_zp)^2 + (X - xp2)^2)^(1/2)))/(2*pi*(Z^2 + (Y - a_yp)^2)^2);
dBz_dz = dBzn_dz + dBzp_dz;
end

== matlab function latest_coil/Inner Coil/Coil 3/MATLAB Function3 ==
  data: X input; Hx_yp output; Y input; Z input; I input; Hy_yp output; Hz_yp output; Hx_yn output; Hy_yn output; Hz_yn output; dBx_dx output; dBx_dy output; dBx_dz output; dBz_dx output; dBz_dy output; dBz_dz output
function [Hx_yp, Hy_yp, Hz_yp, Hx_yn, Hy_yn, Hz_yn, dBx_dx, dBx_dy, dBx_dz, dBz_dx, dBz_dy, dBz_dz] = field_y(X, Y, Z, I)

n = 3;
gy = 440e-6;
gx = 1.475e-3;
gz = 0;
m0 = 4*pi*1e-7;
k = 0.4e-3;
yp1 = -0.6e-3 - (n-1)*k;
yp2 = 0.6e-3 + (n-1)*k;
a_xp = gy;
a_zp = gz;
k_yp = 1./(4*pi*((a_xp-X).^2+(a_zp-Z).^2));
kyp = (yp2-Y)./((yp2-Y).^2+(a_xp-X).^2+(a_zp-Z).^2).^0.5;
k_2yp = (yp1-Y)./((yp1-Y).^2+(a_xp-X).^2+(a_zp-Z).^2).^0.5;

Hx_yp = -((a_zp-Z).*k_yp.*(kyp - k_2yp))*I*m0;
Hy_yp = zeros(size(X,1),size(Y,1),size(Z,1));
Hz_yp = (-(a_xp-X).*k_yp.*(kyp - k_2yp))*I*m0;

a_xn = -gy;
yn1 = -0.8e-3 - (n-1)*k;
yn2 = 0.8e-3 + (n-1)*k;
k_yn = 1./(4*pi*((a_xn-X).^2+(a_zp-Z).^2));
kyn = (yn2-Y)./((yn2-Y).^2+(a_xn-X).^2+(a_zp-Z).^2).^0.5;
k_2yn = (yn1-Y)./((yn1-Y).^2+(a_xn-X).^2+(a_zp-Z).^2).^0.5;

Hx_yn = ((a_zp-Z).*k_yn.*(kyn - k_2yn))*I*m0;
Hy_yn = zeros(size(X,1),size(Y,1),size(Z,1));
Hz_yn = ((a_xn-X).*k_yn.*(kyn - k_2yn))*I*m0;


dBxn_dx = - (I*Z*m0*(((Y - yn1)*(2*X - 2*a_xn))/(2*((X - a_xn)^2 + (Z - a_zp)^2 + (Y - yn1)^2)^(3/2)) - ((Y - yn2)*(2*X - 2*a_xn))/(2*((X - a_xn)^2 + (Z - a_zp)^2 + (Y - yn2)^2)^(3/2))))/(4*pi*((X - a_xn)^2 + (Z - a_zp)^2)) - (I*Z*m0*((Y - yn1)/((X - a_xn)^2 + (Z - a_zp)^2 + (Y - yn1)^2)^(1/2) - (Y - yn2)/((X - a_xn)^2 + (Z - a_zp)^2 + (Y - yn2)^2)^(1/2))*(2*X - 2*a_xn))/(4*pi*((X - a_xn)^2 + (Z - a_zp)^2)^2);
dBxp_dx = (I*Z*m0*(((Y - yp1)*(2*X - 2*a_xp))/(2*((X - a_xp)^2 + (Z - a_zp)^2 + (Y - yp1)^2)^(3/2)) - ((Y - yp2)*(2*X - 2*a_xp))/(2*((X - a_xp)^2 + (Z - a_zp)^2 + (Y - yp2)^2)^(3/2))))/(4*pi*((X - a_xp)^2 + (Z - a_zp)^2)) + (I*Z*m0*((Y - yp1)/((X - a_xp)^2 + (Z - a_zp)^2 + (Y - yp1)^2)^(1/2) - (Y - yp2)/((X - a_xp)^2 + (Z - a_zp)^2 + (Y - yp2)^2)^(1/2))*(2*X - 2*a_xp))/(4*pi*((X - a_xp)^2 + (Z - a_zp)^2)^2);
dBx_dx = dBxp_dx + dBxn_dx;

dBxp_dy = -(I*Z*m0*(1/((X - a_xp)^2 + (Z - a_zp)^2 + (Y - yp1)^2)^(1/2) - 1/((X - a_xp)^2 + (Z - a_zp)^2 + (Y - yp2)^2)^(1/2) - ((Y - yp1)*(2*Y - 2*yp1))/(2*((X - a_xp)^2 + (Z - a_zp)^2 + (Y - yp1)^2)^(3/2)) + ((Y - yp2)*(2*Y - 2*yp2))/(2*((X - a_xp)^2 + (Z - a_zp)^2 + (Y - yp2)^2)^(3/2))))/(4*pi*((X - a_xp)^2 + (Z - a_zp)^2));
dBxn_dy = (I*Z*m0*(1/((X - a_xn)^2 + (Z - a_zp)^2 + (Y - yn1)^2)^(1/2) - 1/((X - a_xn)^2 + (Z - a_zp)^2 + (Y - yn2)^2)^(1/2) - ((Y - yn1)*(2*Y - 2*yn1))/(2*((X - a_xn)^2 + (Z - a_zp)^2 + (Y - yn1)^2)^(3/2)) + ((Y - yn2)*(2*Y - 2*yn2))/(2*((X - a_xn)^2 + (Z - a_zp)^2 + (Y - yn2)^2)^(3/2))))/(4*pi*((X - a_xn)^2 + (Z - a_zp)^2));
dBx_dy = dBxp_dy + dBxn_dy;

dBxp_dz = (I*Z*m0*(((Y - yp1)*(2*Z - 2*a_zp))/(2*((X - a_xp)^2 + (Z - a_zp)^2 + (Y - yp1)^2)^(3/2)) - ((Y - yp2)*(2*Z - 2*a_zp))/(2*((X - a_xp)^2 + (Z - a_zp)^2 + (Y - yp2)^2)^(3/2))))/(4*pi*((X - a_xp)^2 + (Z - a_zp)^2)) - (I*m0*((Y - yp1)/((X - a_xp)^2 + (Z - a_zp)^2 + (Y - yp1)^2)^(1/2) - (Y - yp2)/((X - a_xp)^2 + (Z - a_zp)^2 + (Y - yp2)^2)^(1/2)))/(4*pi*((X - a_xp)^2 + (Z - a_zp)^2)) + (I*Z*m0*((Y - yp1)/((X - a_xp)^2 + (Z - a_zp)^2 + (Y - yp1)^2)^(1/2) - (Y - yp2)/((X - a_xp)^2 + (Z - a_zp)^2 + (Y - yp2)^2)^(1/2))*(2*Z - 2*a_zp))/(4*pi*((X - a_xp)^2 + (Z - a_zp)^2)^2);
dBxn_dz = (I*m0*((Y - yn1)/((X - a_xn)^2 + (Z - a_zp)^2 + (Y - yn1)^2)^(1/2) - (Y - yn2)/((X - a_xn)^2 + (Z - a_zp)^2 + (Y - yn2)^2)^(1/2)))/(4*pi*((X - a_xn)^2 + (Z - a_zp)^2)) - (I*Z*m0*(((Y - yn1)*(2*Z - 2*a_zp))/(2*((X - a_xn)^2 + (Z - a_zp)^2 + (Y - yn1)^2)^(3/2)) - ((Y - yn2)*(2*Z - 2*a_zp))/(2*((X - a_xn)^2 + (Z - a_zp)^2 + (Y - yn2)^2)^(3/2))))/(4*pi*((X - a_xn)^2 + (Z - a_zp)^2)) - (I*Z*m0*((Y - yn1)/((X - a_xn)^2 + (Z - a_zp)^2 + (Y - yn1)^2)^(1/2) - (Y - yn2)/((X - a_xn)^2 + (Z - a_zp)^2 + (Y - yn2)^2)^(1/2))*(2*Z - 2*a_zp))/(4*pi*((X - a_xn)^2 + (Z - a_zp)^2)^2);
dBx_dz = dBxp_dz + dBxn_dz;

dBzn_dx = (I*m0*(X - a_xn)*(((Y - yn1)*(2*X - 2*a_xn))/(2*((X - a_xn)^2 + (Z - a_zp)^2 + (Y - yn1)^2)^(3/2)) - ((Y - yn2)*(2*X - 2*a_xn))/(2*((X - a_xn)^2 + (Z - a_zp)^2 + (Y - yn2)^2)^(3/2))))/(4*pi*(Z^2 + (X - a_xn)^2)) - (I*m0*((Y - yn1)/((X - a_xn)^2 + (Z - a_zp)^2 + (Y - yn1)^2)^(1/2) - (Y - yn2)/((X - a_xn)^2 + (Z - a_zp)^2 + (Y - yn2)^2)^(1/2)))/(4*pi*(Z^2 + (X - a_xn)^2)) + (I*m0*((Y - yn1)/((X - a_xn)^2 + (Z - a_zp)^2 + (Y - yn1)^2)^(1/2) - (Y - yn2)/((X - a_xn)^2 + (Z - a_zp)^2 + (Y - yn2)^2)^(1/2))*(X - a_xn)*(2*X - 2*a_xn))/(4*pi*(Z^2 + (X - a_xn)^2)^2);
dBzp_dx = (I*m0*((Y - yp1)/((X - a_xp)^2 + (Z - a_zp)^2 + (Y - yp1)^2)^(1/2) - (Y - yp2)/((X - a_xp)^2 + (Z - a_zp)^2 + (Y - yp2)^2)^(1/2)))/(4*pi*(Z^2 + (X - a_xp)^2)) - (I*m0*(X - a_xp)*(((Y - yp1)*(2*X - 2*a_xp))/(2*((X - a_xp)^2 + (Z - a_zp)^2 + (Y - yp1)^2)^(3/2)) - ((Y - yp2)*(2*X - 2*a_xp))/(2*((X - a_xp)^2 + (Z - a_zp)^2 + (Y - yp2)^2)^(3/2))))/(4*pi*(Z^2 + (X - a_xp)^2)) - (I*m0*((Y - yp1)/((X - a_xp)^2 + (Z - a_zp)^2 + (Y - yp1)^2)^(1/2) - (Y - yp2)/((X - a_xp)^2 + (Z - a_zp)^2 + (Y - yp2)^2)^(1/2))*(X - a_xp)*(2*X - 2*a_xp))/(4*pi*(Z^2 + (X - a_xp)^2)^2);
dBz_dx = dBzp_dx + dBzn_dx;

dBzn_dy = -(I*m0*(X - a_xn)*(1/((X - a_xn)^2 + (Z - a_zp)^2 + (Y - yn1)^2)^(1/2) - 1/((X - a_xn)^2 + (Z - a_zp)^2 + (Y - yn2)^2)^(1/2) - ((Y - yn1)*(2*Y - 2*yn1))/(2*((X - a_xn)^2 + (Z - a_zp)^2 + (Y - yn1)^2)^(3/2)) + ((Y - yn2)*(2*Y - 2*yn2))/(2*((X - a_xn)^2 + (Z - a_zp)^2 + (Y - yn2)^2)^(3/2))))/(4*pi*(Z^2 + (X - a_xn)^2));
dBzp_dy = (I*m0*(X - a_xp)*(1/((X - a_xp)^2 + (Z - a_zp)^2 + (Y - yp1)^2)^(1/2) - 1/((X - a_xp)^2 + (Z - a_zp)^2 + (Y - yp2)^2)^(1/2) - ((Y - yp1)*(2*Y - 2*yp1))/(2*((X - a_xp)^2 + (Z - a_zp)^2 + (Y - yp1)^2)^(3/2)) + ((Y - yp2)*(2*Y - 2*yp2))/(2*((X - a_xp)^2 + (Z - a_zp)^2 + (Y - yp2)^2)^(3/2))))/(4*pi*(Z^2 + (X - a_xp)^2));
dBz_dy = dBzn_dy + dBzp_dy;

dBzn_dz = (I*m0*(X - a_xn)*(((Y - yn1)*(2*Z - 2*a_zp))/(2*((X - a_xn)^2 + (Z - a_zp)^2 + (Y - yn1)^2)^(3/2)) - ((Y - yn2)*(2*Z - 2*a_zp))/(2*((X - a_xn)^2 + (Z - a_zp)^2 + (Y - yn2)^2)^(3/2))))/(4*pi*(Z^2 + (X - a_xn)^2)) + (I*Z*m0*((Y - yn1)/((X - a_xn)^2 + (Z - a_zp)^2 + (Y - yn1)^2)^(1/2) - (Y - yn2)/((X - a_xn)^2 + (Z - a_zp)^2 + (Y - yn2)^2)^(1/2))*(X - a_xn))/(2*pi*(Z^2 + (X - a_xn)^2)^2);
dBzp_dz = - (I*m0*(X - a_xp)*(((Y - yp1)*(2*Z - 2*a_zp))/(2*((X - a_xp)^2 + (Z - a_zp)^2 + (Y - yp1)^2)^(3/2)) - ((Y - yp2)*(2*Z - 2*a_zp))/(2*((X - a_xp)^2 + (Z - a_zp)^2 + (Y - yp2)^2)^(3/2))))/(4*pi*(Z^2 + (X - a_xp)^2)) - (I*Z*m0*((Y - yp1)/((X - a_xp)^2 + (Z - a_zp)^2 + (Y - yp1)^2)^(1/2) - (Y - yp2)/((X - a_xp)^2 + (Z - a_zp)^2 + (Y - yp2)^2)^(1/2))*(X - a_xp))/(2*pi*(Z^2 + (X - a_xp)^2)^2);
dBz_dz = dBzn_dz + dBzp_dz;
end

== matlab function latest_coil/Inner Coil/Coil 3/MATLAB Function4 ==
  data: Hx_xp input; Hy_xp input; Hz_xp input; Hx output; Hx_xn input; Hy_xn input; Hy output; Hz output; Hz_xn input; Hx_yp input; Hy_yp input; Hz_yp input; Hx_yn input; Hy_yn input; Hz_yn input
function [Hx, Hy, Hz] = field_sum(Hx_xp, Hy_xp, Hz_xp, Hx_xn, Hy_xn, Hz_xn, Hx_yp, Hy_yp, Hz_yp, Hx_yn, Hy_yn, Hz_yn)
Hx = Hx_xp + Hx_xn + Hx_yp + Hx_yn;
Hy = Hy_xp + Hy_xn + Hy_yp + Hy_yn;
Hz = Hz_xp + Hz_xn + Hz_yp + Hz_yn;
end

== matlab function latest_coil/Inner Coil/Coil 4/MATLAB Function ==
  data: X input; Hx_xp output; Y input; Z input; I input; Hy_xp output; Hz_xp output; Hx_xn output; Hy_xn output; Hz_xn output; dBy_dx output; dBy_dy output; dBy_dz output; dBz_dx output; dBz_dy output; dBz_dz output
function [Hx_xp, Hy_xp, Hz_xp, Hx_xn, Hy_xn, Hz_xn,dBy_dx ,dBy_dy, dBy_dz, dBz_dx ,dBz_dy, dBz_dz] = field_x(X, Y, Z, I)
n = 4;
% gy = 430e-6;
gz = 0;
gx = 1.875e-3;
m0 = 4*pi*1e-7;
k = 0.4e-3;
xp1 = -0.8e-3 - (n-1)*k;
xp2 = 0.8e-3 + (n-1)*k;
a_yp = gx; 
a_zp = gz;
k_p = 1./(4*pi*((a_yp-Y).^2+(a_zp-Z).^2));
kxp = (xp2-X)./((xp2-X).^2+(a_yp-Y).^2+(a_zp-Z).^2).^0.5;
k_2xp = (xp1-X)./((xp1-X).^2+(a_yp-Y).^2+(a_zp-Z).^2).^0.5;

Hx_xp = zeros(size(X,1),size(Y,1),size(Z,1));
Hy_xp = (-(a_zp-Z).*k_p.*(kxp - k_2xp))*I*m0;
Hz_xp = (-(a_yp-Y).*k_p.*(kxp - k_2xp))*I*m0;

a_yn = -gx;
xn1 = -1e-3 - (n-1)*k;
xn2 = 1e-3 + (n-1)*k;
k_n = 1./(4*pi*((a_yn-Y).^2+(a_zp-Z).^2));
kxn = (xn2-X)./((xn2-X).^2+(a_yn-Y).^2+(a_zp-Z).^2).^0.5;
k_2xn = (xn1-X)./((xn1-X).^2+(a_yn-Y).^2+(a_zp-Z).^2).^0.5;

Hx_xn = zeros(size(X,1),size(Y,1),size(Z,1));
Hy_xn = ((a_zp-Z).*k_n.*(kxn - k_2xn))*I*m0;
Hz_xn = ((a_yn-Y).*k_n.*(kxn - k_2xn))*I*m0;

dByn_dx = (I*Z*m0*(1/((Y - a_yn)^2 + (Z - a_zp)^2 + (X - xn1)^2)^(1/2) - 1/((Y - a_yn)^2 + (Z - a_zp)^2 + (X - xn2)^2)^(1/2) - ((X - xn1)*(2*X - 2*xn1))/(2*((Y - a_yn)^2 + (Z - a_zp)^2 + (X - xn1)^2)^(3/2)) + ((X - xn2)*(2*X - 2*xn2))/(2*((Y - a_yn)^2 + (Z - a_zp)^2 + (X - xn2)^2)^(3/2))))/(4*pi*((Y - a_yn)^2 + (Z - a_zp)^2));
dByp_dx = -(I*Z*m0*(1/((Y - a_yp)^2 + (Z - a_zp)^2 + (X - xp1)^2)^(1/2) - 1/((Y - a_yp)^2 + (Z - a_zp)^2 + (X - xp2)^2)^(1/2) - ((X - xp1)*(2*X - 2*xp1))/(2*((Y - a_yp)^2 + (Z - a_zp)^2 + (X - xp1)^2)^(3/2)) + ((X - xp2)*(2*X - 2*xp2))/(2*((Y - a_yp)^2 + (Z - a_zp)^2 + (X - xp2)^2)^(3/2))))/(4*pi*((Y - a_yp)^2 + (Z - a_zp)^2));
dBy_dx = dByp_dx + dByn_dx;

dByp_dy = (I*Z*m0*(((X - xp1)*(2*Y - 2*a_yp))/(2*((Y - a_yp)^2 + (Z - a_zp)^2 + (X - xp1)^2)^(3/2)) - ((X - xp2)*(2*Y - 2*a_yp))/(2*((Y - a_yp)^2 + (Z - a_zp)^2 + (X - xp2)^2)^(3/2))))/(4*pi*((Y - a_yp)^2 + (Z - a_zp)^2)) + (I*Z*m0*(2*Y - 2*a_yp)*((X - xp1)/((Y - a_yp)^2 + (Z - a_zp)^2 + (X - xp1)^2)^(1/2) - (X - xp2)/((Y - a_yp)^2 + (Z - a_zp)^2 + (X - xp2)^2)^(1/2)))/(4*pi*((Y - a_yp)^2 + (Z - a_zp)^2)^2);
dByn_dy = - (I*Z*m0*(((X - xn1)*(2*Y - 2*a_yn))/(2*((Y - a_yn)^2 + (Z - a_zp)^2 + (X - xn1)^2)^(3/2)) - ((X - xn2)*(2*Y - 2*a_yn))/(2*((Y - a_yn)^2 + (Z - a_zp)^2 + (X - xn2)^2)^(3/2))))/(4*pi*((Y - a_yn)^2 + (Z - a_zp)^2)) - (I*Z*m0*(2*Y - 2*a_yn)*((X - xn1)/((Y - a_yn)^2 + (Z - a_zp)^2 + (X - xn1)^2)^(1/2) - (X - xn2)/((Y - a_yn)^2 + (Z - a_zp)^2 + (X - xn2)^2)^(1/2)))/(4*pi*((Y - a_yn)^2 + (Z - a_zp)^2)^2);
dBy_dy = dByp_dy + dByn_dy;

dByp_dz = (I*Z*m0*(((X - xp1)*(2*Z - 2*a_zp))/(2*((Y - a_yp)^2 + (Z - a_zp)^2 + (X - xp1)^2)^(3/2)) - ((X - xp2)*(2*Z - 2*a_zp))/(2*((Y - a_yp)^2 + (Z - a_zp)^2 + (X - xp2)^2)^(3/2))))/(4*pi*((Y - a_yp)^2 + (Z - a_zp)^2)) - (I*m0*((X - xp1)/((Y - a_yp)^2 + (Z - a_zp)^2 + (X - xp1)^2)^(1/2) - (X - xp2)/((Y - a_yp)^2 + (Z - a_zp)^2 + (X - xp2)^2)^(1/2)))/(4*pi*((Y - a_yp)^2 + (Z - a_zp)^2)) + (I*Z*m0*(2*Z - 2*a_zp)*((X - xp1)/((Y - a_yp)^2 + (Z - a_zp)^2 + (X - xp1)^2)^(1/2) - (X - xp2)/((Y - a_yp)^2 + (Z - a_zp)^2 + (X - xp2)^2)^(1/2)))/(4*pi*((Y - a_yp)^2 + (Z - a_zp)^2)^2);
dByn_dz = (I*m0*((X - xn1)/((Y - a_yn)^2 + (Z - a_zp)^2 + (X - xn1)^2)^(1/2) - (X - xn2)/((Y - a_yn)^2 + (Z - a_zp)^2 + (X - xn2)^2)^(1/2)))/(4*pi*((Y - a_yn)^2 + (Z - a_zp)^2)) - (I*Z*m0*(((X - xn1)*(2*Z - 2*a_zp))/(2*((Y - a_yn)^2 + (Z - a_zp)^2 + (X - xn1)^2)^(3/2)) - ((X - xn2)*(2*Z - 2*a_zp))/(2*((Y - a_yn)^2 + (Z - a_zp)^2 + (X - xn2)^2)^(3/2))))/(4*pi*((Y - a_yn)^2 + (Z - a_zp)^2)) - (I*Z*m0*(2*Z - 2*a_zp)*((X - xn1)/((Y - a_yn)^2 + (Z - a_zp)^2 + (X - xn1)^2)^(1/2) - (X - xn2)/((Y - a_yn)^2 + (Z - a_zp)^2 + (X - xn2)^2)^(1/2)))/(4*pi*((Y - a_yn)^2 + (Z - a_zp)^2)^2);
dBy_dz = dByp_dz + dByn_dz;

dBzp_dx = (I*m0*(Y - a_yp)*(1/((Y - a_yp)^2 + (Z - a_zp)^2 + (X - xp1)^2)^(1/2) - 1/((Y - a_yp)^2 + (Z - a_zp)^2 + (X - xp2)^2)^(1/2) - ((X - xp1)*(2*X - 2*xp1))/(2*((Y - a_yp)^2 + (Z - a_zp)^2 + (X - xp1)^2)^(3/2)) + ((X - xp2)*(2*X - 2*xp2))/(2*((Y - a_yp)^2 + (Z - a_zp)^2 + (X - xp2)^2)^(3/2))))/(4*pi*(Z^2 + (Y - a_yp)^2));
dBzn_dx = -(I*m0*(Y - a_yn)*(1/((Y - a_yn)^2 + (Z - a_zp)^2 + (X - xn1)^2)^(1/2) - 1/((Y - a_yn)^2 + (Z - a_zp)^2 + (X - xn2)^2)^(1/2) - ((X - xn1)*(2*X - 2*xn1))/(2*((Y - a_yn)^2 + (Z - a_zp)^2 + (X - xn1)^2)^(3/2)) + ((X - xn2)*(2*X - 2*xn2))/(2*((Y - a_yn)^2 + (Z - a_zp)^2 + (X - xn2)^2)^(3/2))))/(4*pi*(Z^2 + (Y - a_yn)^2));
dBz_dx = dBzp_dx + dBzn_dx;

dBzn_dy = (I*m0*(Y - a_yn)*(((X - xn1)*(2*Y - 2*a_yn))/(2*((Y - a_yn)^2 + (Z - a_zp)^2 + (X - xn1)^2)^(3/2)) - ((X - xn2)*(2*Y - 2*a_yn))/(2*((Y - a_yn)^2 + (Z - a_zp)^2 + (X - xn2)^2)^(3/2))))/(4*pi*(Z^2 + (Y - a_yn)^2)) - (I*m0*((X - xn1)/((Y - a_yn)^2 + (Z - a_zp)^2 + (X - xn1)^2)^(1/2) - (X - xn2)/((Y - a_yn)^2 + (Z - a_zp)^2 + (X - xn2)^2)^(1/2)))/(4*pi*(Z^2 + (Y - a_yn)^2)) + (I*m0*(Y - a_yn)*(2*Y - 2*a_yn)*((X - xn1)/((Y - a_yn)^2 + (Z - a_zp)^2 + (X - xn1)^2)^(1/2) - (X - xn2)/((Y - a_yn)^2 + (Z - a_zp)^2 + (X - xn2)^2)^(1/2)))/(4*pi*(Z^2 + (Y - a_yn)^2)^2);
dBzp_dy = (I*m0*((X - xp1)/((Y - a_yp)^2 + (Z - a_zp)^2 + (X - xp1)^2)^(1/2) - (X - xp2)/((Y - a_yp)^2 + (Z - a_zp)^2 + (X - xp2)^2)^(1/2)))/(4*pi*(Z^2 + (Y - a_yp)^2)) - (I*m0*(Y - a_yp)*(((X - xp1)*(2*Y - 2*a_yp))/(2*((Y - a_yp)^2 + (Z - a_zp)^2 + (X - xp1)^2)^(3/2)) - ((X - xp2)*(2*Y - 2*a_yp))/(2*((Y - a_yp)^2 + (Z - a_zp)^2 + (X - xp2)^2)^(3/2))))/(4*pi*(Z^2 + (Y - a_yp)^2)) - (I*m0*(Y - a_yp)*(2*Y - 2*a_yp)*((X - xp1)/((Y - a_yp)^2 + (Z - a_zp)^2 + (X - xp1)^2)^(1/2) - (X - xp2)/((Y - a_yp)^2 + (Z - a_zp)^2 + (X - xp2)^2)^(1/2)))/(4*pi*(Z^2 + (Y - a_yp)^2)^2);
dBz_dy = dBzn_dy + dBzp_dy;

dBzn_dz = (I*m0*(Y - a_yn)*(((X - xn1)*(2*Z - 2*a_zp))/(2*((Y - a_yn)^2 + (Z - a_zp)^2 + (X - xn1)^2)^(3/2)) - ((X - xn2)*(2*Z - 2*a_zp))/(2*((Y - a_yn)^2 + (Z - a_zp)^2 + (X - xn2)^2)^(3/2))))/(4*pi*(Z^2 + (Y - a_yn)^2)) + (I*Z*m0*(Y - a_yn)*((X - xn1)/((Y - a_yn)^2 + (Z - a_zp)^2 + (X - xn1)^2)^(1/2) - (X - xn2)/((Y - a_yn)^2 + (Z - a_zp)^2 + (X - xn2)^2)^(1/2)))/(2*pi*(Z^2 + (Y - a_yn)^2)^2);
dBzp_dz = - (I*m0*(Y - a_yp)*(((X - xp1)*(2*Z - 2*a_zp))/(2*((Y - a_yp)^2 + (Z - a_zp)^2 + (X - xp1)^2)^(3/2)) - ((X - xp2)*(2*Z - 2*a_zp))/(2*((Y - a_yp)^2 + (Z - a_zp)^2 + (X - xp2)^2)^(3/2))))/(4*pi*(Z^2 + (Y - a_yp)^2)) - (I*Z*m0*(Y - a_yp)*((X - xp1)/((Y - a_yp)^2 + (Z - a_zp)^2 + (X - xp1)^2)^(1/2) - (X - xp2)/((Y - a_yp)^2 + (Z - a_zp)^2 + (X - xp2)^2)^(1/2)))/(2*pi*(Z^2 + (Y - a_yp)^2)^2);
dBz_dz = dBzn_dz + dBzp_dz;
end

== matlab function latest_coil/Inner Coil/Coil 4/MATLAB Function3 ==
  data: X input; Hx_yp output; Y input; Z input; I input; Hy_yp output; Hz_yp output; Hx_yn output; Hy_yn output; Hz_yn output; dBx_dx output; dBx_dy output; dBx_dz output; dBz_dx output; dBz_dy output; dBz_dz output
function [Hx_yp, Hy_yp, Hz_yp, Hx_yn, Hy_yn, Hz_yn, dBx_dx, dBx_dy, dBx_dz, dBz_dx, dBz_dy, dBz_dz] = field_y(X, Y, Z, I)

n = 4;
gy = 430e-6;
% gx = 1.875e-3;
gz = 0;
m0 = 4*pi*1e-7;
k = 0.4e-3;
yp1 = -0.6e-3 - (n-1)*k;
yp2 = 0.6e-3 + (n-1)*k;
a_xp = gy;
a_zp = gz;
k_yp = 1./(4*pi*((a_xp-X).^2+(a_zp-Z).^2));
kyp = (yp2-Y)./((yp2-Y).^2+(a_xp-X).^2+(a_zp-Z).^2).^0.5;
k_2yp = (yp1-Y)./((yp1-Y).^2+(a_xp-X).^2+(a_zp-Z).^2).^0.5;

Hx_yp = -((a_zp-Z).*k_yp.*(kyp - k_2yp))*I*m0;
Hy_yp = zeros(size(X,1),size(Y,1),size(Z,1));
Hz_yp = (-(a_xp-X).*k_yp.*(kyp - k_2yp))*I*m0;

a_xn = -gy;
yn1 = -0.8e-3 - (n-1)*k;
yn2 = 0.8e-3 + (n-1)*k;
k_yn = 1./(4*pi*((a_xn-X).^2+(a_zp-Z).^2));
kyn = (yn2-Y)./((yn2-Y).^2+(a_xn-X).^2+(a_zp-Z).^2).^0.5;
k_2yn = (yn1-Y)./((yn1-Y).^2+(a_xn-X).^2+(a_zp-Z).^2).^0.5;

Hx_yn = ((a_zp-Z).*k_yn.*(kyn - k_2yn))*I*m0;
Hy_yn = zeros(size(X,1),size(Y,1),size(Z,1));
Hz_yn = ((a_xn-X).*k_yn.*(kyn - k_2yn))*I*m0;

dBxn_dx = - (I*Z*m0*(((Y - yn1)*(2*X - 2*a_xn))/(2*((X - a_xn)^2 + (Z - a_zp)^2 + (Y - yn1)^2)^(3/2)) - ((Y - yn2)*(2*X - 2*a_xn))/(2*((X - a_xn)^2 + (Z - a_zp)^2 + (Y - yn2)^2)^(3/2))))/(4*pi*((X - a_xn)^2 + (Z - a_zp)^2)) - (I*Z*m0*((Y - yn1)/((X - a_xn)^2 + (Z - a_zp)^2 + (Y - yn1)^2)^(1/2) - (Y - yn2)/((X - a_xn)^2 + (Z - a_zp)^2 + (Y - yn2)^2)^(1/2))*(2*X - 2*a_xn))/(4*pi*((X - a_xn)^2 + (Z - a_zp)^2)^2);
dBxp_dx = (I*Z*m0*(((Y - yp1)*(2*X - 2*a_xp))/(2*((X - a_xp)^2 + (Z - a_zp)^2 + (Y - yp1)^2)^(3/2)) - ((Y - yp2)*(2*X - 2*a_xp))/(2*((X - a_xp)^2 + (Z - a_zp)^2 + (Y - yp2)^2)^(3/2))))/(4*pi*((X - a_xp)^2 + (Z - a_zp)^2)) + (I*Z*m0*((Y - yp1)/((X - a_xp)^2 + (Z - a_zp)^2 + (Y - yp1)^2)^(1/2) - (Y - yp2)/((X - a_xp)^2 + (Z - a_zp)^2 + (Y - yp2)^2)^(1/2))*(2*X - 2*a_xp))/(4*pi*((X - a_xp)^2 + (Z - a_zp)^2)^2);
dBx_dx = dBxp_dx + dBxn_dx;

dBxp_dy = -(I*Z*m0*(1/((X - a_xp)^2 + (Z - a_zp)^2 + (Y - yp1)^2)^(1/2) - 1/((X - a_xp)^2 + (Z - a_zp)^2 + (Y - yp2)^2)^(1/2) - ((Y - yp1)*(2*Y - 2*yp1))/(2*((X - a_xp)^2 + (Z - a_zp)^2 + (Y - yp1)^2)^(3/2)) + ((Y - yp2)*(2*Y - 2*yp2))/(2*((X - a_xp)^2 + (Z - a_zp)^2 + (Y - yp2)^2)^(3/2))))/(4*pi*((X - a_xp)^2 + (Z - a_zp)^2));
dBxn_dy = (I*Z*m0*(1/((X - a_xn)^2 + (Z - a_zp)^2 + (Y - yn1)^2)^(1/2) - 1/((X - a_xn)^2 + (Z - a_zp)^2 + (Y - yn2)^2)^(1/2) - ((Y - yn1)*(2*Y - 2*yn1))/(2*((X - a_xn)^2 + (Z - a_zp)^2 + (Y - yn1)^2)^(3/2)) + ((Y - yn2)*(2*Y - 2*yn2))/(2*((X - a_xn)^2 + (Z - a_zp)^2 + (Y - yn2)^2)^(3/2))))/(4*pi*((X - a_xn)^2 + (Z - a_zp)^2));
dBx_dy = dBxp_dy + dBxn_dy;

dBxp_dz = (I*Z*m0*(((Y - yp1)*(2*Z - 2*a_zp))/(2*((X - a_xp)^2 + (Z - a_zp)^2 + (Y - yp1)^2)^(3/2)) - ((Y - yp2)*(2*Z - 2*a_zp))/(2*((X - a_xp)^2 + (Z - a_zp)^2 + (Y - yp2)^2)^(3/2))))/(4*pi*((X - a_xp)^2 + (Z - a_zp)^2)) - (I*m0*((Y - yp1)/((X - a_xp)^2 + (Z - a_zp)^2 + (Y - yp1)^2)^(1/2) - (Y - yp2)/((X - a_xp)^2 + (Z - a_zp)^2 + (Y - yp2)^2)^(1/2)))/(4*pi*((X - a_xp)^2 + (Z - a_zp)^2)) + (I*Z*m0*((Y - yp1)/((X - a_xp)^2 + (Z - a_zp)^2 + (Y - yp1)^2)^(1/2) - (Y - yp2)/((X - a_xp)^2 + (Z - a_zp)^2 + (Y - yp2)^2)^(1/2))*(2*Z - 2*a_zp))/(4*pi*((X - a_xp)^2 + (Z - a_zp)^2)^2);
dBxn_dz = (I*m0*((Y - yn1)/((X - a_xn)^2 + (Z - a_zp)^2 + (Y - yn1)^2)^(1/2) - (Y - yn2)/((X - a_xn)^2 + (Z - a_zp)^2 + (Y - yn2)^2)^(1/2)))/(4*pi*((X - a_xn)^2 + (Z - a_zp)^2)) - (I*Z*m0*(((Y - yn1)*(2*Z - 2*a_zp))/(2*((X - a_xn)^2 + (Z - a_zp)^2 + (Y - yn1)^2)^(3/2)) - ((Y - yn2)*(2*Z - 2*a_zp))/(2*((X - a_xn)^2 + (Z - a_zp)^2 + (Y - yn2)^2)^(3/2))))/(4*pi*((X - a_xn)^2 + (Z - a_zp)^2)) - (I*Z*m0*((Y - yn1)/((X - a_xn)^2 + (Z - a_zp)^2 + (Y - yn1)^2)^(1/2) - (Y - yn2)/((X - a_xn)^2 + (Z - a_zp)^2 + (Y - yn2)^2)^(1/2))*(2*Z - 2*a_zp))/(4*pi*((X - a_xn)^2 + (Z - a_zp)^2)^2);
dBx_dz = dBxp_dz + dBxn_dz;

dBzn_dx = (I*m0*(X - a_xn)*(((Y - yn1)*(2*X - 2*a_xn))/(2*((X - a_xn)^2 + (Z - a_zp)^2 + (Y - yn1)^2)^(3/2)) - ((Y - yn2)*(2*X - 2*a_xn))/(2*((X - a_xn)^2 + (Z - a_zp)^2 + (Y - yn2)^2)^(3/2))))/(4*pi*(Z^2 + (X - a_xn)^2)) - (I*m0*((Y - yn1)/((X - a_xn)^2 + (Z - a_zp)^2 + (Y - yn1)^2)^(1/2) - (Y - yn2)/((X - a_xn)^2 + (Z - a_zp)^2 + (Y - yn2)^2)^(1/2)))/(4*pi*(Z^2 + (X - a_xn)^2)) + (I*m0*((Y - yn1)/((X - a_xn)^2 + (Z - a_zp)^2 + (Y - yn1)^2)^(1/2) - (Y - yn2)/((X - a_xn)^2 + (Z - a_zp)^2 + (Y - yn2)^2)^(1/2))*(X - a_xn)*(2*X - 2*a_xn))/(4*pi*(Z^2 + (X - a_xn)^2)^2);
dBzp_dx = (I*m0*((Y - yp1)/((X - a_xp)^2 + (Z - a_zp)^2 + (Y - yp1)^2)^(1/2) - (Y - yp2)/((X - a_xp)^2 + (Z - a_zp)^2 + (Y - yp2)^2)^(1/2)))/(4*pi*(Z^2 + (X - a_xp)^2)) - (I*m0*(X - a_xp)*(((Y - yp1)*(2*X - 2*a_xp))/(2*((X - a_xp)^2 + (Z - a_zp)^2 + (Y - yp1)^2)^(3/2)) - ((Y - yp2)*(2*X - 2*a_xp))/(2*((X - a_xp)^2 + (Z - a_zp)^2 + (Y - yp2)^2)^(3/2))))/(4*pi*(Z^2 + (X - a_xp)^2)) - (I*m0*((Y - yp1)/((X - a_xp)^2 + (Z - a_zp)^2 + (Y - yp1)^2)^(1/2) - (Y - yp2)/((X - a_xp)^2 + (Z - a_zp)^2 + (Y - yp2)^2)^(1/2))*(X - a_xp)*(2*X - 2*a_xp))/(4*pi*(Z^2 + (X - a_xp)^2)^2);
dBz_dx = dBzp_dx + dBzn_dx;

dBzn_dy = -(I*m0*(X - a_xn)*(1/((X - a_xn)^2 + (Z - a_zp)^2 + (Y - yn1)^2)^(1/2) - 1/((X - a_xn)^2 + (Z - a_zp)^2 + (Y - yn2)^2)^(1/2) - ((Y - yn1)*(2*Y - 2*yn1))/(2*((X - a_xn)^2 + (Z - a_zp)^2 + (Y - yn1)^2)^(3/2)) + ((Y - yn2)*(2*Y - 2*yn2))/(2*((X - a_xn)^2 + (Z - a_zp)^2 + (Y - yn2)^2)^(3/2))))/(4*pi*(Z^2 + (X - a_xn)^2));
dBzp_dy = (I*m0*(X - a_xp)*(1/((X - a_xp)^2 + (Z - a_zp)^2 + (Y - yp1)^2)^(1/2) - 1/((X - a_xp)^2 + (Z - a_zp)^2 + (Y - yp2)^2)^(1/2) - ((Y - yp1)*(2*Y - 2*yp1))/(2*((X - a_xp)^2 + (Z - a_zp)^2 + (Y - yp1)^2)^(3/2)) + ((Y - yp2)*(2*Y - 2*yp2))/(2*((X - a_xp)^2 + (Z - a_zp)^2 + (Y - yp2)^2)^(3/2))))/(4*pi*(Z^2 + (X - a_xp)^2));
dBz_dy = dBzn_dy + dBzp_dy;

dBzn_dz = (I*m0*(X - a_xn)*(((Y - yn1)*(2*Z - 2*a_zp))/(2*((X - a_xn)^2 + (Z - a_zp)^2 + (Y - yn1)^2)^(3/2)) - ((Y - yn2)*(2*Z - 2*a_zp))/(2*((X - a_xn)^2 + (Z - a_zp)^2 + (Y - yn2)^2)^(3/2))))/(4*pi*(Z^2 + (X - a_xn)^2)) + (I*Z*m0*((Y - yn1)/((X - a_xn)^2 + (Z - a_zp)^2 + (Y - yn1)^2)^(1/2) - (Y - yn2)/((X - a_xn)^2 + (Z - a_zp)^2 + (Y - yn2)^2)^(1/2))*(X - a_xn))/(2*pi*(Z^2 + (X - a_xn)^2)^2);
dBzp_dz = - (I*m0*(X - a_xp)*(((Y - yp1)*(2*Z - 2*a_zp))/(2*((X - a_xp)^2 + (Z - a_zp)^2 + (Y - yp1)^2)^(3/2)) - ((Y - yp2)*(2*Z - 2*a_zp))/(2*((X - a_xp)^2 + (Z - a_zp)^2 + (Y - yp2)^2)^(3/2))))/(4*pi*(Z^2 + (X - a_xp)^2)) - (I*Z*m0*((Y - yp1)/((X - a_xp)^2 + (Z - a_zp)^2 + (Y - yp1)^2)^(1/2) - (Y - yp2)/((X - a_xp)^2 + (Z - a_zp)^2 + (Y - yp2)^2)^(1/2))*(X - a_xp))/(2*pi*(Z^2 + (X - a_xp)^2)^2);
dBz_dz = dBzn_dz + dBzp_dz;
end

== matlab function latest_coil/Inner Coil/Coil 4/MATLAB Function4 ==
  data: Hx_xp input; Hy_xp input; Hz_xp input; Hx output; Hx_xn input; Hy_xn input; Hy output; Hz output; Hz_xn input; Hx_yp input; Hy_yp input; Hz_yp input; Hx_yn input; Hy_yn input; Hz_yn input
function [Hx, Hy, Hz] = field_sum(Hx_xp, Hy_xp, Hz_xp, Hx_xn, Hy_xn, Hz_xn, Hx_yp, Hy_yp, Hz_yp, Hx_yn, Hy_yn, Hz_yn)
Hx = Hx_xp + Hx_xn + Hx_yp + Hx_yn;
Hy = Hy_xp + Hy_xn + Hy_yp + Hy_yn;
Hz = Hz_xp + Hz_xn + Hz_yp + Hz_yn;
end
